simulink model "ch4f30"  (Simulink 3.00)
settings: Solver=ode45  SolverMode=SingleTasking  StartTime=0.0  StopTime=25  RelTol=1e-3  AbsTol=1e-6
CloseFcn:
  | ;slview('closediagram',bdroot);
settings Model: OptimizeBlockIOStorage=off

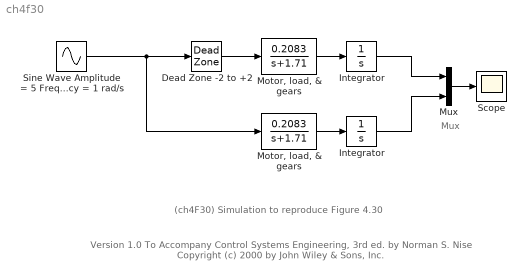
== system ch4f30 ==
  note: Mux
  note: (ch4F30) Simulation to reproduce Figure 4.30
  note: Version 1.0
      | To Accompany Control Systems Engineering, 3rd ed. by Norman S. Nise
      | Copyright (c) 2000 by John Wiley & Sons, Inc.
  Dead Zone -2 to +2 : DeadZone  LowerValue=-2  UpperValue=2
  Integrator : Integrator  ExternalReset=none  InitialConditionSource=internal  InitialCondition=0  LimitOutput=off  UpperSaturationLimit=inf  LowerSaturationLimit=-inf  ShowSaturationPort=off  ShowStatePort=off  AbsoluteTolerance=auto
  "Integrator " : Integrator  ExternalReset=none  InitialConditionSource=internal  InitialCondition=0  LimitOutput=off  UpperSaturationLimit=inf  LowerSaturationLimit=-inf  ShowSaturationPort=off  ShowStatePort=off  AbsoluteTolerance=auto
  "Motor, load, & gears" : TransferFcn  Numerator=0.2083  Denominator=[1 1.71]
  "Motor, load, & gears " : TransferFcn  Numerator=0.2083  Denominator=[1 1.71]
  Mux : Mux  Inputs=2
  Scope : Scope
      settings: TickLabels=on  TimeRange=25  YMin=0  YMax=1.2  SaveToWorkspace=off  SaveName=ScopeData  DataFormat=Matrix
  Sine Wave Amplitude = 5 Frequency = 1 rad/s : Sin  Amplitude=5  Frequency=1  Phase=0  SampleTime=0
  wires:
  Sine Wave Amplitude = 5 Frequency = 1 rad/s/1 -> "Motor, load, & gears "/1, Dead Zone -2 to +2/1
  "Motor, load, & gears"/1 -> Integrator/1
  "Motor, load, & gears "/1 -> "Integrator "/1
  Integrator/1 -> Mux/1
  Dead Zone -2 to +2/1 -> "Motor, load, & gears"/1
  "Integrator "/1 -> Mux/2
  Mux/1 -> Scope/1
